simulink model "Char_After_Balancing_by_Mean_3S1P"  (R2024b)
settings: Solver=VariableStepAuto  StartTime=0.0  StopTime=3000  RelTol=1e-3
undefined symbols (not defined in the file): Ion, Lithium
libraries: spsCurrentMeasurementLib x5, spsSeriesRLCBranchLib x4, spsVoltageMeasurementLib x4, spsBatteryLib x3, spsMosfetLib x3, spsIdealSwitchLib x2, spsDCVoltageSourceLib x1, sps_lib x1
settings Model: Creator=HP
settings SolverCC: ZeroCrossAlgorithm=Adaptive
settings DebuggingCC: IgnoredZcDiagnostic=none
settings RTWCC: GPUComputeCapability=3.5

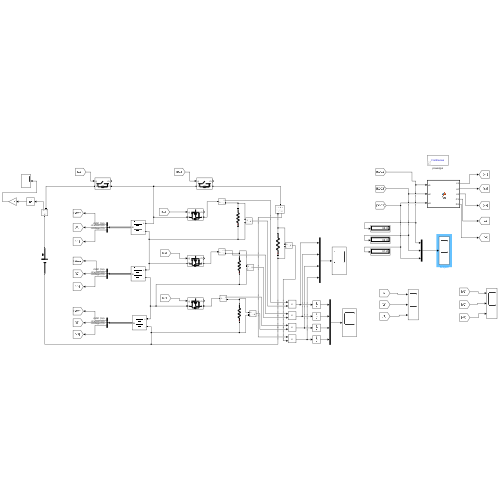
[thumbnail: Simulink's stored preview of the top-level diagram]
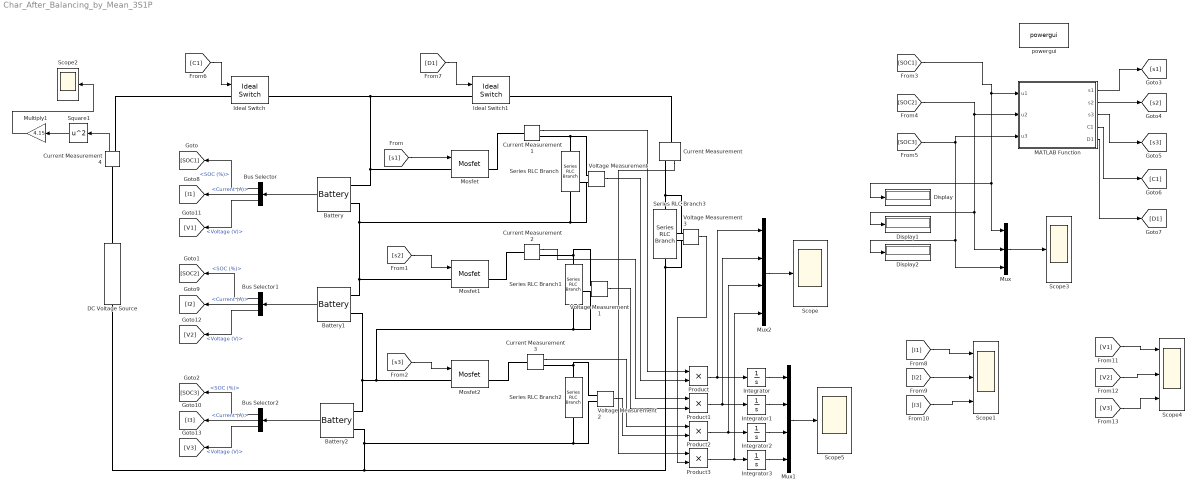
== system Char_After_Balancing_by_Mean_3S1P ==
  Battery : spsBatteryLib/Battery  BatType=Lithium-Ion  NomV=3.6  NomQ=2.6  SOC=70  Batt_Tr=1  PresetModel=on  MaxQ=2.6  MinV=2.7  FullV=4.1904  Dis_rate=1.1304  R=0.013846  Normal_OP=2.3513  expZone="[3.8894     0.12774]"
  Battery1 : spsBatteryLib/Battery  BatType=Lithium-Ion  NomV=3.6  NomQ=2.6  SOC=60  Batt_Tr=1  PresetModel=on  MaxQ=2.6  MinV=2.7  FullV=4.1904  Dis_rate=1.1304  R=0.013846  Normal_OP=2.3513  expZone="[3.8894     0.12774]"
  Battery2 : spsBatteryLib/Battery  BatType=Lithium-Ion  NomV=3.6  NomQ=2.6  SOC=50  Batt_Tr=10  PresetModel=on  MaxQ=2.6  MinV=2.7  FullV=4.1904  Dis_rate=1.1304  R=0.013846  Normal_OP=2.3513  expZone="[3.8894     0.12774]"
  Bus Selector : BusSelector  OutputSignals=SOC (%),Current (A),Voltage (V)
  Bus Selector1 : BusSelector  OutputSignals=SOC (%),Current (A),Voltage (V)
  Bus Selector2 : BusSelector  OutputSignals=SOC (%),Current (A),Voltage (V)
  Current Measurement{,1..4} (5 alike) : spsCurrentMeasurementLib/Current Measurement  PhasorSimulation=off  OutputType=Complex  PSBequivalent=0
  DC Voltage Source : spsDCVoltageSourceLib/DC Voltage Source  Amplitude=12  Measurements=None
  Display : Display
  Display1 : Display
  Display2 : Display
  Ideal Switch : spsIdealSwitchLib/Ideal Switch  Ron=0.001  Lon=0  IC=0  Rs=1e5  Cs=inf  Measurements=on
  Ideal Switch1 : spsIdealSwitchLib/Ideal Switch  Ron=0.001  Lon=0  IC=0  Rs=1e5  Cs=inf  Measurements=on
  Integrator{,1..3} (4 alike) : Integrator
  MATLAB Function : MATLAB Function  TreatAsAtomicUnit=on
  Mosfet : spsMosfetLib/Mosfet  Ron=0.1  Lon=0  Rd=0.01  Vfd=0  IC=0  Rs=1e5  Cs=inf  Measurements=on
  Mosfet1 : spsMosfetLib/Mosfet  Ron=0.1  Lon=0  Rd=0.01  Vfd=0  IC=0  Rs=1e5  Cs=inf  Measurements=on
  Mosfet2 : spsMosfetLib/Mosfet  Ron=0.1  Lon=0  Rd=0.01  Vfd=0  IC=0  Rs=1e5  Cs=inf  Measurements=on
  Multiply1 : Gain  Gain=4.15
  Mux : Mux  Inputs=3
  Mux1 : Mux
  Mux2 : Mux
  Product{,1..3} (4 alike) : Product
  Scope{,2..3,5} (4 alike) : Scope
  Scope1 : Scope  NumInputPorts=3
  Scope4 : Scope  NumInputPorts=3
  Series RLC Branch : spsSeriesRLCBranchLib/Series RLC Branch  LConnTagsString=__new0  RConnTagsString=__new0  BranchType=R  Resistance=1.3  Inductance=1e-3  SetiL0=off  InitialCurrent=0  Capacitance=1e-6  Setx0=off  InitialVoltage=0  Measurements=None
  Series RLC Branch1 : spsSeriesRLCBranchLib/Series RLC Branch  LConnTagsString=__new0  RConnTagsString=__new0  BranchType=R  Resistance=1.3  Inductance=1e-3  SetiL0=off  InitialCurrent=0  Capacitance=1e-6  Setx0=off  InitialVoltage=0  Measurements=None
  Series RLC Branch2 : spsSeriesRLCBranchLib/Series RLC Branch  LConnTagsString=__new0  RConnTagsString=__new0  BranchType=R  Resistance=1.3  Inductance=1e-3  SetiL0=off  InitialCurrent=0  Capacitance=1e-6  Setx0=off  InitialVoltage=0  Measurements=None
  Series RLC Branch3 : spsSeriesRLCBranchLib/Series RLC Branch  LConnTagsString=__new0  RConnTagsString=__new0  BranchType=R  Resistance=4.15  Inductance=1e-3  SetiL0=off  InitialCurrent=0  Capacitance=1e-6  Setx0=off  InitialVoltage=0  Measurements=None
  Square1 : Math  Operator=square
  Voltage Measurement{,1..3} (4 alike) : spsVoltageMeasurementLib/Voltage Measurement  PhasorSimulation=off  OutputType=Complex  PSBequivalent=0
  powergui : sps_lib/powergui  Priority=1  SimulationMode=Continuous  SampleTime=50e-6  frequency=60  Iterations=50  frequencyindice=0  Pbase=100e6  ErrMax=1e-4  UnitsV=kV  UnitsW=MW  buscounter=0  FunctionMessages=off  echomessages=off  EnableUseOfTLC=off  CurrentSourceSwitches=off  DisableSnubberDevices=off  DisableRonSwitches=off  DisableVfSwitches=off  DisplayEquations=off  AutomaticDiscreteSolvers=off  SolverType=Tustin/Backward Euler (TBE)  Interpol=off  ExternalGateDelay=off  methode=off  Ts=100  x0status=blocks  SPID=on  SwTol=0  HookPort=off  NonlinearTolerance=1e-4  nMaxIteration=100  ContinueOnMaxIteration=off  RestoreLinks=warning  ResistiveCurrentMeasurement=off  Frange=[0:2:500]  Ylog=off  Xlog=on  ShowGrid=off  save=off  variable=ZData  structure=0  ZoomFFT=off  StartTime=0.0  cycles=1  DisplayStyle=1  fundamental=60  FreqAxis=off  MaxFrequency=1000  frequencyindicesteady=1  RmsSteady=1  display=off
  wires:
  Battery/1 -> Bus Selector/1
  Battery1/1 -> Bus Selector1/1
  Battery2/1 -> Bus Selector2/1
  Bus Selector/1 -> [SOC1]  "<SOC (%)>"
  Bus Selector1/1 -> [SOC2]  "<SOC (%)>"
  Bus Selector2/1 -> [SOC3]  "<SOC (%)>"
  [SOC1] -> Mux/1, Display/1, MATLAB Function/1(u1)
  [SOC2] -> Display1/1, Mux/2, MATLAB Function/2(u2)
  [SOC3] -> Mux/3, Display2/1, MATLAB Function/3(u3)
  MATLAB Function/1(s1) -> [s1]
  MATLAB Function/2(s2) -> [s2]
  MATLAB Function/3(s3) -> [s3]
  Mux/1 -> Scope3/1
  [s1] -> Mosfet/1
  [s2] -> Mosfet1/1
  [s3] -> Mosfet2/1
  Bus Selector/2 -> [I1]  "<Current (A)>"
  Bus Selector/3 -> [V1]  "<Voltage (V)>"
  Bus Selector1/2 -> [I2]  "<Current (A)>"
  Bus Selector1/3 -> [V2]  "<Voltage (V)>"
  Bus Selector2/2 -> [I3]  "<Current (A)>"
  Bus Selector2/3 -> [V3]  "<Voltage (V)>"
  [I2] -> Scope1/2
  [I1] -> Scope1/1
  [I3] -> Scope1/3
  [V2] -> Scope4/2
  [V1] -> Scope4/1
  [V3] -> Scope4/3
  [C1] -> Ideal Switch/1
  [D1] -> Ideal Switch1/1
  MATLAB Function/4(C1) -> [C1]
  MATLAB Function/5(D1) -> [D1]
  Current Measurement4/1 -> Square1/1
  Square1/1 -> Multiply1/1
  Multiply1/1 -> Scope2/1
  Current Measurement1/1 -> Product/1
  Voltage Measurement/1 -> Product/2
  Current Measurement2/1 -> Product1/1
  Voltage Measurement1/1 -> Product1/2
  Current Measurement3/1 -> Product2/1
  Voltage Measurement2/1 -> Product2/2
  Current Measurement/1 -> Product3/1
  Voltage Measurement3/1 -> Product3/2
  Product/1 -> Mux2/1, Integrator/1
  Product1/1 -> Integrator1/1, Mux2/2
  Product2/1 -> Integrator2/1, Mux2/3
  Product3/1 -> Mux2/4, Integrator3/1
  Integrator/1 -> Mux1/1
  Integrator1/1 -> Mux1/2
  Integrator2/1 -> Mux1/3
  Integrator3/1 -> Mux1/4
  Mux1/1 -> Scope5/1
  Mux2/1 -> Scope/1
  connections:
  Battery/LConn2 -- Series RLC Branch/LConn1 -- Voltage Measurement/LConn2 -- Mosfet1/LConn1 -- Battery1/LConn1
  Series RLC Branch1/LConn1 -- Battery2/LConn1 -- Battery1/LConn2 -- Mosfet2/LConn1 -- Voltage Measurement1/LConn2
  Voltage Measurement2/LConn2 -- Series RLC Branch2/LConn1 -- Battery2/LConn2 -- Voltage Measurement3/LConn2 -- Series RLC Branch3/LConn1 -- DC Voltage Source/LConn1
  Ideal Switch/RConn1 -- Ideal Switch1/LConn1 -- Battery/LConn1 -- Mosfet/LConn1
  Ideal Switch1/RConn1 -- Current Measurement/LConn1
  Current Measurement/RConn1 -- Series RLC Branch3/RConn1 -- Voltage Measurement3/LConn1
  Current Measurement1/LConn1 -- Mosfet/RConn1
  Current Measurement2/LConn1 -- Mosfet1/RConn1
  Current Measurement3/LConn1 -- Mosfet2/RConn1
  Series RLC Branch2/RConn1 -- Current Measurement3/RConn1 -- Voltage Measurement2/LConn1
  Series RLC Branch/RConn1 -- Current Measurement1/RConn1 -- Voltage Measurement/LConn1
  Series RLC Branch1/RConn1 -- Current Measurement2/RConn1 -- Voltage Measurement1/LConn1
  Current Measurement4/LConn1 -- DC Voltage Source/RConn1
  Current Measurement4/RConn1 -- Ideal Switch/LConn1

== matlab function Char_After_Balancing_by_Mean_3S1P/MATLAB Function ==
  data: u1 input; s1 output; u2 input; u3 input; s2 output; s3 output; C1 output; D1 output
function [s1,s2,s3,C1,D1]  = fcn(u1,u2,u3)
u1 = int32(u1);
u2 = int32(u2);
u3 = int32(u3);

mean = (u1+u2+u3)/3;

if(u1>mean)
    
      s1 = 1;
else
      s1 = 0;  

end
if(u2>mean)
    
      s2 = 1;
else
      s2 = 0;  

end
if(u3>mean)
    
      s3 = 1;
else
      s3 = 0;  

end

if((u1==u2)||(u2==u3))
    D1=0;
    C1=1;
else
    D1=0;
    C1=0;
end
